simulink model "position_control"  (R2021a)
settings: Solver=ode23t  StartTime=0.0  StopTime=200  RelTol=1e-5
values from neighbouring files (symbols this model uses):
  g = 9.81    [quad_params.m]
  I = [     0.005831943165131                   0                   0 ... (first row only)    [quad_params.m]
  Kd_rates = [0.05,0.05,0.1]'    [quad_params.m]
  Kd_vel = [0.8,0.8,0.3]'    [quad_params.m]
  Ki_vel = [0.1,0.1,0.1]'    [quad_params.m]
  km = 1.2e-7    (= 1.2e-07)    [quad_params.m]
  Kp_att = [6,6,6]'    [quad_params.m]
  Kp_pos = [7,7,3]'    [quad_params.m]
  Kp_rates = [10,10,10]'    [quad_params.m]
  Kp_vel = [3,3,5]'    [quad_params.m]
  kt = 0.9e-5    (= 9e-06)    [quad_params.m]
  L = 0.2    [quad_params.m]
  m = 0.9272    [quad_params.m]
  q_init = [1;0;0;0]    [quad_params.m]
  rate_p_max = 3.5    [quad_params.m]
  thrust_max = thrust_max_per_motor*4    (= 32)    [quad_params.m]
  thrust_max_per_motor = 8    [quad_params.m]
  tilt_max = pi/6    (= 0.523598775598)    [quad_params.m]
  TQ_max_per_motor = km*(w_max.^2)    [quad_params.m]
  Vb_init = [0;0;0]    [quad_params.m]
  vel_xy_max = 15    [quad_params.m]
  vel_z_max = 10    [quad_params.m]
  wb_init = [0;0;0]    [quad_params.m]
  Xe_init = [0;0;0]    [quad_params.m]
undefined symbols (not defined in the file or in its folder): pm_0, sigbuilder_block, Vm_0, X, xme_0, Y, Z
libraries: simulink_extras x16, nesl_utility x5, aerolibutil x4, sm_lib x4, simulink x3, pid_lib x3, sharedtransform x3, sharedutil x1, vrlib x1, aerolibanim x1
(part 3 of 3)

== system position_control/Trajectory command/Yaw Sine/yaw ==
  Demux : Demux  Tag=STV Demux
      settings: DisplayOption=none
  FromWs : FromWorkspace  Tag=STV FromWs  VariableName=tuvar
      SigBuilderData=|
      | common.afterFinalStr = 'Extrapolate'
      | common.sampleTime = 0
      | dataSet(1).timeRange = [0 200]
      | dataSet(1).name = 'small_steps'
      | dataSet(2).timeRange = [0 200]
      | dataSet(2).name = 'zStairs_xyConstVEL'
      | dataSet(3).timeRange = [0 500]
      | dataSet(3).name = 'sineWaves'
      | dataSet(4).timeRange = [0 200]
      | dataSet(4).name = 'ZERO'
      | dataSet(5).timeRange = [0 200]
      | dataSet(5).name = 'SEARCH_P1'
      | sbobj.Name = 'Signal Builder'
      | sbobj.Groups(1).Name = 'small_steps'
      | sbobj.Groups(1).Signals(1).Name = 'Z'
      | sbobj.Groups(1).Signals(1).XData = [0 10 10.000001 20 20.000001 30 30.000001 55 200]
      | sbobj.Groups(1).Signals(1).YData = [0 0 2 2 2 2 2 2 2]
      | sbobj.Groups(1).Signals(2).Name = 'Y'
      | sbobj.Groups(1).Signals(2).XData = [0 10 10.000001 20 20.000001 30 30.000001 55 200]
      | sbobj.Groups(1).Signals(2).YData = [0 0 0 0 3 3 3 3 3]
      | sbobj.Groups(1).Signals(3).Name = 'X'
      | sbobj.Groups(1).Signals(3).XData = [0 10 10.000001 20 20.000001 30 30.000001 55 200]
      | sbobj.Groups(1).Signals(3).YData = [0 0 0 0 0 0 1 1 1]
      | sbobj.Groups(1).Signals(4).Name = 'Yaw'
      | sbobj.Groups(1).Signals(4).XData = [0 200]
      | sbobj.Groups(1).Signals(4).YData = [0 0]
      | sbobj.Groups(1).TimeRange = [0 200]
      | sbobj.Groups(2).Name = 'zStairs_xyConstVEL'
      | sbobj.Groups(2).Signals(1).Name = 'Z'
      | sbobj.Groups(2).Signals(1).XData = [0 10 10.000001 20 20.000001 30 30.000001 40 40.000001 55 200]
      | sbobj.Groups(2).Signals(1).YData = [0 0 1 1 2 2 1 1 0 0 0]
      | sbobj.Groups(2).Signals(2).Name = 'Y'
      | sbobj.Groups(2).Signals(2).XData = [0 10 10.000001 20 20.000001 30 30.000001 40 40.000001 55 200]
      | sbobj.Groups(2).Signals(2).YData = [0 1 1.0000001 2 2.0000001 3 3.0000001 4 4.0000001 5.5 20]
      | sbobj.Groups(2).Signals(3).Name = 'X'
      | sbobj.Groups(2).Signals(3).XData = [0 10 10.000001 20 20.000001 30 30.000001 40 40.000001 55 200]
      | sbobj.Groups(2).Signals(3).YData = [0 0.5 0.50000005 1 1.00000005 1.5 1.50000005 2 2.00000005 2.75 10]
      | sbobj.Groups(2).Signals(4).Name = 'Yaw'
      | sbobj.Groups(2).Signals(4).XData = [0 200]
      | sbobj.Groups(2).Signals(4).YData = [0 0]
      | sbobj.Groups(2).TimeRange = [0 200]
      | sbobj.Groups(3).Name = 'sineWaves'
      | sbobj.Groups(3).Signals(1).Name = 'Z'
      | sbobj.Groups(3).Signals(1).XData = [0 0.1 0.2 0.3 0.4 0.5 0.6 0.7 0.8 0.9 1 1.1 ... (5001 elements, 1x5001)]
      | sbobj.Groups(3).Signals(1).YData = [0 0.0314107325553 0.0627904665622 0.0941082340641 0.125333128258 0.156434333994 0.18738115819 0.218143060119 0.248689681547 0.278990876699 0.309016742004 0.338737645607 ... (5001 elements, 1x5001)]
      | sbobj.Groups(3).Signals(2).Name = 'Y'
      | sbobj.Groups(3).Signals(2).XData = [0 0.1 0.2 0.3 0.4 0.5 0.6 0.7 0.8 0.9 1 1.1 ... (5001 elements, 1x5001)]
      | sbobj.Groups(3).Signals(2).YData = [0 0.01 0.02 0.03 0.04 0.05 0.06 0.07 0.08 0.09 0.1 0.11 ... (5001 elements, 1x5001)]
      | sbobj.Groups(3).Signals(3).Name = 'X'
      | sbobj.Groups(3).Signals(3).XData = [0 0.1 0.2 0.3 0.4 0.5 0.6 0.7 0.8 0.9 1 1.1 ... (5001 elements, 1x5001)]
      | sbobj.Groups(3).Signals(3).YData = [0 0.0157073040455 0.0314107325553 0.04710641095 0.0627904665622 0.0784590295926 0.0941082340641 0.109734218776 0.125333128258 0.140901113717 0.156434333994 0.171928956505 ... (5001 elements, 1x5001)]
      | sbobj.Groups(3).Signals(4).Name = 'Yaw'
      | sbobj.Groups(3).Signals(4).XData = [0 500]
      | sbobj.Groups(3).Signals(4).YData = [0 0]
      | sbobj.Groups(3).TimeRange = [0 500]
      | sbobj.Groups(4).Name = 'ZERO'
      | sbobj.Groups(4).Signals(1).Name = 'Z'
      | sbobj.Groups(4).Signals(1).XData = [0 200]
      | sbobj.Groups(4).Signals(1).YData = [0 0]
      | sbobj.Groups(4).Signals(2).Name = 'Y'
      | sbobj.Groups(4).Signals(2).XData = [0 200]
      | sbobj.Groups(4).Signals(2).YData = [0 0]
      | sbobj.Groups(4).Signals(3).Name = 'X'
      | sbobj.Groups(4).Signals(3).XData = [0 200]
      | sbobj.Groups(4).Signals(3).YData = [0 0]
      | sbobj.Groups(4).Signals(4).Name = 'Yaw'
      | sbobj.Groups(4).Signals(4).XData = [0 200]
      | sbobj.Groups(4).Signals(4).YData = [0 0]
      | sbobj.Groups(4).TimeRange = [0 200]
      | sbobj.Groups(5).Name = 'SEARCH_P1'
      | sbobj.Groups(5).Signals(1).Name = 'Z'
      | sbobj.Groups(5).Signals(1).XData = [0 9.9 200]
      | sbobj.Groups(5).Signals(1).YData = [0 0 0]
      | sbobj.Groups(5).Signals(2).Name = 'Y'
      | sbobj.Groups(5).Signals(2).XData = [0 200]
      | sbobj.Groups(5).Signals(2).YData = [0 0]
      | sbobj.Groups(5).Signals(3).Name = 'X'
      | sbobj.Groups(5).Signals(3).XData = [0 200]
      | sbobj.Groups(5).Signals(3).YData = [0 0]
      | sbobj.Groups(5).Signals(4).Name = 'Yaw'
      | sbobj.Groups(5).Signals(4).XData = [0 0.689655172414 1.37931034483 2.06896551724 2.75862068966 3.44827586207 4.13793103448 4.8275862069 5.51724137931 6.20689655172 6.89655172414 7.58620689655 ... (291 elements, 1x291)]
      | sbobj.Groups(5).Signals(4).YData = [0 0.644911320633 1.25966730468 1.81552264558 2.28648616538 2.65053613334 2.89064997756 2.99560024155 2.96047956762 2.78693015945 2.48306699447 2.06309837656 ... (291 elements, 1x291)]
      | sbobj.Groups(5).TimeRange = [0 200]
  Z : Outport  VectorParamsAs1DForOutWhenUnconnected=off
  Y : Outport  Tag=STV Outport  Port=2  VectorParamsAs1DForOutWhenUnconnected=off
  X : Outport  Tag=STV Outport  Port=3  VectorParamsAs1DForOutWhenUnconnected=off
  Yaw : Outport  Tag=STV Outport  Port=4
  wires:
  Demux/4 -> Yaw/1
  Demux/3 -> X/1
  Demux/2 -> Y/1
  FromWs/1 -> Demux/1
  Demux/1 -> Z/1

== system position_control/Control allocation and motor control/Ideal Actuators with allocation/Control allocation/Subsystem ==
  w_per_sec : Inport
  Constant3 : Constant  Value=3.141592653589793
  Gain1 : Gain  Gain=2
  Product : Product  Inputs=*/
  RPS : Outport
  wires:
  Gain1/1 -> Product/2  "2PI"
  w_per_sec/1 -> Product/1
  Constant3/1 -> Gain1/1
  Product/1 -> RPS/1

== system position_control/Control allocation and motor control/Ideal Actuators with allocation/Control allocation/W2_checker ==
  w2_CMD : Inport
  Assertion{,1..3} (4 alike) : Assertion
  Compare To Constant : simulink/Logic and Bit Operations/Compare To Constant  relop=>=  const=0  OutDataTypeStr=boolean
  Demux : Demux
  w2 : Outport  VectorParamsAs1DForOutWhenUnconnected=off
  wires:
  w2_CMD/1 -> w2/1, Compare To Constant/1
  Compare To Constant/1 -> Demux/1
  Demux/1 -> Assertion/1
  Demux/4 -> Assertion3/1
  Demux/3 -> Assertion2/1
  Demux/2 -> Assertion1/1

== system position_control/Control allocation and motor control/Ideal Actuators with allocation/Perfect actuators/Motor Control ==
  w_CMD : Inport
  Demux : Demux
  Mux : Mux
  w CMD vs Actual : Scope  NumInputPorts=4
  w_MUX : Subsystem
  w : Outport  VectorParamsAs1DForOutWhenUnconnected=off
  wires:
  Demux/4 -> Mux/4
  Demux/3 -> Mux/3
  Demux/2 -> Mux/2
  Demux/1 -> Mux/1
  w_CMD/1 -> [W_CMD], Demux/1
  w_MUX/4(w4) -> w CMD vs Actual/4
  w_MUX/2(w2) -> w CMD vs Actual/2
  w_MUX/3(w3) -> w CMD vs Actual/3
  w_MUX/1(w1) -> w CMD vs Actual/1
  [W_CMD] -> w_MUX/1(W_CMD)
  Mux/1 -> w_MUX/2(W), w/1

== system position_control/Quad_EOM/Integrate_quaternion/NORMLIZE_occasionally/Adjust_to_UNITY ==
  note: Every 10 seconds normalize
      | the quaternion to ensure it is a
      | UNIT quaternion
  qin : Inport
  Data Type Conversion : DataTypeConversion  OutDataTypeStr=double
  Detect Increase : simulink/Logic and Bit Operations/Detect Increase  vinit=0.0  OutDataTypeStr=boolean
  MATLAB Function : MATLAB Function  TreatAsAtomicUnit=on
  Pulse Generator : DiscretePulseGenerator  PulseType=Time based  Period=10  PulseWidth=50
  Scope : Scope
  q_unit : Outport
  wires:
  Pulse Generator/1 -> Detect Increase/1
  Detect Increase/1 -> Data Type Conversion/1
  MATLAB Function/1(q) -> q_unit/1
  Data Type Conversion/1 -> MATLAB Function/1(change_signal)
  qin/1 -> MATLAB Function/2(q_in)
  MATLAB Function/2(mag_of_q) -> Scope/1

== system position_control/Control allocation and motor control/Ideal Actuators with allocation/Perfect actuators/Motor Control/w_MUX ==
  W_CMD : Inport
  W : Inport  Port=2
  Demux1 : Demux
  Demux2 : Demux
  Mux{,1..3} (4 alike) : Mux  Inputs=2
  w1 : Outport  VectorParamsAs1DForOutWhenUnconnected=off
  w2 : Outport  Port=2  VectorParamsAs1DForOutWhenUnconnected=off
  w3 : Outport  Port=3  VectorParamsAs1DForOutWhenUnconnected=off
  w4 : Outport  Port=4  VectorParamsAs1DForOutWhenUnconnected=off
  wires:
  W_CMD/1 -> Demux2/1
  W/1 -> Demux1/1
  Mux/1 -> w1/1
  Mux1/1 -> w2/1
  Mux3/1 -> w4/1
  Mux2/1 -> w3/1
  Demux2/1 -> Mux/1
  Demux2/2 -> Mux1/1
  Demux2/3 -> Mux2/1
  Demux2/4 -> Mux3/1
  Demux1/1 -> Mux/2
  Demux1/2 -> Mux1/2
  Demux1/3 -> Mux2/2
  Demux1/4 -> Mux3/2

== matlab function position_control/Quad_EOM/Integrate_quaternion/MATLAB Function2 ==
  data: R input; phi output; theta output; psi output
function [phi,theta,psi] = euler_from_rot(R)
% Get Euler angles from rotation matrix (wolrd to body rotation matrix)
%NOTE:  this is bRg ... and NOT gRb

phi   = atan2(R(2,3),R(3,3));
theta = -asin(R(1,3));
psi   = atan2(R(1,2), R(1,1));
end

== matlab function position_control/Thrust to attitude/Subsystem/MATLAB Function3 ==
  data: acc_w input size=[2 1]; phi_cmd output size=[2 1]; g input size=[1 1]; yaw_cmd input; theta_cmd output
function [phi_cmd,theta_cmd]= acc2ang(acc_w, g,yaw_cmd)
    
    phi_cmd = 1/g*(acc_w(1)*sin(yaw_cmd)-acc_w(2)*cos(yaw_cmd));
    theta_cmd = 1/g*(acc_w(1)*cos(yaw_cmd)+acc_w(2)*sin(yaw_cmd));
end

== matlab function position_control/Control allocation and motor control/Ideal Actuators with allocation/Perfect actuators/Allocation matrix (motor speed to twist) ==
  data: L input; Thrust output; kt input; km input; w2_col input; M_x output; M_y output; M_z output
function [Thrust, M_x, M_y, M_z] = mixer(L, kt, km, w2_col)
%#codegen



    % construct the co-efficient matrix:
    %  T = C * w^2
    
%     C = [
%         kt  ,   kt   ,   kt  ,   kt  ;
%         0   , -L*kt  ,   0   , L*kt  ;
%        L*kt ,   0    , -L*kt ,   0   ;
%         km ,   -km   ,  km  ,   -km  ;
%     ];

    C = [
        -kt  ,   -kt  ,   -kt ,   -kt  ;
        0    , -L*kt   ,   0   , L*kt  ;
       L*kt ,   0    , -L*kt  ,   0   ;
        -km  ,   km   ,  -km  ,   km  ;
    ];

    % solve for the FM_col
    %   FM_col = [Thrust, M_x, M_y, M_z].' ;
    
    FM_col  =  C * w2_col;
    
    Thrust  =  FM_col(1);
    M_x     =  FM_col(2);
    M_y     =  FM_col(3);
    M_z     =  FM_col(4);
    
end

== matlab function position_control/Quad_EOM/Integrate_quaternion/calc_bRg ==
  data: q input double size=[4, 1]; bRg output double size=[3 3]
function bRg = quat2dcm(q)
% convert quaternion to DCM
% the DCM represent coordinate transformation of a vector in inertial axes
% into body axes (bRg)

% VERY SLOW in SIMULINK

    q0    = q(1);
    qx    = q(2);
    qy    = q(3);
    qz    = q(4);
    
    C_11  = qx^2 + q0^2 - qy^2 - qz^2;
    C_12  = 2*(qx*qy + qz*q0);
    C_13  = 2*(qx*qz - qy*q0);
       
    C_21  = 2*(qx*qy - qz*q0);
    C_22  = qy^2 + q0^2 - qx^2 - qz^2;
    C_23  = 2*(qy*qz + qx*q0);
    
    C_31  = 2*(qx*qz + qy*q0);
    C_32  = 2*(qy*qz - qx*q0);
    C_33  = qz^2 + q0^2 - qx^2 - qy^2;
    
    
    bRg = [ C_11, C_12, C_13;
            C_21, C_22, C_23;
            C_31, C_32, C_33;   ];   


end

== matlab function position_control/Quad_EOM/Integrate_quaternion/calc_q_DOT ==
  data: q input double size=[4, 1]; q_dot output double size=[4 1]; wb input double size=[3, 1]
function q_dot = q_dot_from_rates(q, wb)
% angular rates are related to quaternion derivative by:
% note: this transformation is in body-fixed frame (body rates and
% quaternion in body-fixed frame)
% q_dot  = 0.5 * W^T * wb;
% 
% W = 
%    [-q1,  q0,  q3, -q2]
%    [-q2, -q3,  q0,  q1]
%    [-q3,  q2, -q1,  q0]
% W_transpose = 
%             [-q1, -q2, -q3]
%             [ q0, -q3,  q2]
%             [ q3,  q0, -q1]
%             [-q2,  q1,  q0]

q0     = q(1);
q1     = q(2);
q2     = q(3);
q3     = q(4);

W_transpose =  [
                 -q1, -q2, -q3;
                  q0, -q3,  q2;
                  q3,  q0, -q1;
                 -q2,  q1,  q0;
                 ];

wb = wb(:);

q_dot  = 0.5 * W_transpose * wb;

end

== matlab function position_control/Thrust to attitude/Subsystem/MATLAB Function5 ==
  data: body_z input; thr_dir output; acc_sp input; g input; hover_thrust input; thr_mag output
function [thr_dir,thr_mag] = project_thrust(body_z,acc_sp,g, hover_thrust)
    % body_z is normalized acceleration pointing down
    % hover_thrust = m*g
    collective_thrust = acc_sp(3) * (hover_thrust/g) - hover_thrust; % T=(m*acc_cmd)-(mg)
	% Project thrust to planned body attitude
    tmp = dot([0,0,1]',body_z);
	collective_thrust = collective_thrust./tmp;
	thr_dir = body_z*collective_thrust;

    % thrust body setpoint is the norm of the thrust vector
    thr_mag = norm(thr_dir);
    
%     final_body_z = unit(body_z); % normalize body_z
%     
%     % vector of desired yaw direction in XY plane, rotated by PI/2
%     y_c = [-sin(yaw_sp), cos(yaw_sp), 0.0].';
%     % desired body_x axis, orthogonal to body_z
% 	body_x = cross(y_c,final_body_z);
%     
%    % keep nose to front while inverted upside down
% 	if (final_body_z(3) < 0.0
% 		body_x = -body_x;
%     end
%     body_x = unit(body_x); % normalize body_x
%     % desired body_y axis
%     body_y = mod(final_body_z,body_x);
%     
%     % fill rotation matrix and convert to quaternion
%     world_unit = [0,0,1]';
%     body_unit = body_z;
%     dot_product_unit = dot(body_unit,world_unit);
% 	angle = acos(dot_product_unit);
%     body_unit = cos(angle) * world_unit + sin(angle) * body_unit;

== matlab function position_control/Thrust to attitude/Subsystem/MATLAB Function6 ==
  data: acc_w input size=[2 1]; u1_thrust output size=[2 1]; g input size=[1 1]; m input
function u1_thrust = acc2thrust(acc_w, g,m)
    
    u1_thrust = m*g+acc_w(3);
end

== matlab function position_control/Quad_EOM/Integrate_quaternion/NORMLIZE_occasionally/Adjust_to_UNITY/MATLAB Function ==
  data: change_signal input double size=1; q output; q_in input double size=[4 1]; mag_of_q output
function [q, mag_of_q] = fcn(change_signal, q_in)

if(change_signal > 0.5)
    q = q_in / norm(q_in);
else
    q = q_in;
end

mag_of_q = norm(q);

end

== matlab function position_control/Thrust to attitude/Subsystem/MATLAB Function7 ==
  data: acc_w input size=[2 1]; phi_cmd output size=[2 1]; g input size=[1 1]; yaw_cmd input; theta_cmd output
function [phi_cmd,theta_cmd]= acc2ang(acc_w, g,yaw_cmd)
    
    phi_cmd = 1/g*(acc_w(1)*sin(yaw_cmd)-acc_w(2)*cos(yaw_cmd));
    theta_cmd = 1/g*(acc_w(1)*cos(yaw_cmd)+acc_w(2)*sin(yaw_cmd));
end

== matlab function position_control/Thrust to attitude/Subsystem/MATLAB Function8 ==
  data: thrust_vec input; q_sp output; heading_angle input
function q_sp = thrust2quat(thrust_vec,heading_angle)
% full attitude control using both thrust vector and desired yaw
    % inputs: thrust_vec, heading_angle
    % extracted from: ardupilot
    thrust_vec_unit = [0,0,1]';
    
    if norm(thrust_vec)^2<1e-15
        thrust_vec = thrust_vec_unit;
    else
        thrust_vec = unit(thrust_vec);  % or normalize(thrust_vec)
    end
    % the cross product of the desired and target thrust vector defines the rotation vector
    thrust_vec_cross = cross(thrust_vec_unit, thrust_vec);
    % the dot product is used to calculate the angle between the target and desired thrust vectors
    thrust_vec_angle = acos(dot(thrust_vec_unit, thrust_vec));
    % Normalize the thrust rotation vector
    thrust_vec_length = norm(thrust_vec_cross);
    if thrust_vec_length==0 
        thrust_vec_length = 1;
        thrust_vec_cross = thrust_vec_unit;
    end
    thrust_vec_dir = thrust_vec_cross/thrust_vec_length;
    
    % convert thrust_vec_cross and thrust_vec_angle to quaternion
    thrust_vec_quat = axang2quat([thrust_vec_dir.', thrust_vec_angle]);
    % yaw quaternion from heading_angle and [0,0,1]
    yaw_quat = axang2quat([[0.0, 0.0, 1.0], heading_angle]);
    
    % multiple both quats to get quat setpoint
    q_sp = quatmultiply(thrust_vec_quat,yaw_quat);

== matlab function position_control/Attitude control/MATLAB Function1 ==
  data: q0 input; y output
function y = sign(q0)
if q0>=0
    y = 1;
else
    y = -1;
end

== matlab function position_control/Control allocation and motor control/Ideal Actuators with allocation/Control allocation/FM_to_w2 ==
  data: L input; w2_cmd output; kt input; km input; Thrust input; M_x input; M_y input; M_z input
function w2_cmd = control_allocation(L, kt, km, Thrust, M_x, M_y, M_z)
%#codegen

    % construct the co-efficient matrix:
    %  F_and_M = C * w^2
    %
    % C = [
    %     kt  ,   kt   ,   kt  ,   kt  ;
    %     0   , -L*kt  ,   0   , L*kt  ;
    %    L*kt ,   0    , -L*kt ,   0   ;
    %     km ,   -km   ,  km  ,   -km  ;
    % ];

    % used Symbolic toolbox to compute inv(C)
%     C_inv = [
%                 1/(4*kt),          0 ,  1/(2*L*kt),  1/(4*km);
%                 1/(4*kt), -1/(2*L*kt),           0,  -1/(4*km); 
%                 1/(4*kt),          0 , -1/(2*L*kt),  1/(4*km);
%                 1/(4*kt), 1/(2*L*kt) ,          0 ,  -1/(4*km);
%              ];
         
    C_inv = [
             -1/(4*kt),            0,   1/(2*L*kt), -1/(4*km);
             -1/(4*kt),  -1/(2*L*kt),            0,  1/(4*km);
             -1/(4*kt),            0,  -1/(2*L*kt), -1/(4*km);
             -1/(4*kt),   1/(2*L*kt),            0,  1/(4*km);
            ];        
    % solve for the w^2 vec
    F_and_M_col = [Thrust, M_x, M_y, M_z].' ;

    w2_cmd = C_inv * F_and_M_col;
   
end

== matlab function position_control/Position+Velocity Control/Velocity PID Controller/MATLAB Function ==
  data: Tmax input; tilt_max input; Tx input; Tx output; Ty input; Tz input; Ty output
function [Tx, Ty] = limit_tilt( Tmax, tilt_max, Tx, Ty, Tz)
% horizontal thrust magnituide at max tilt angle
T_hor = abs(Tz)*tan(tilt_max);
% maximum availble horizontal thrust magnituide 
T_hor_max = sqrt(abs(Tmax^2-Tz^2));
% limit horizontal thrust magnituide to max available
T_hor = min(T_hor,T_hor_max);

% saturate horizonal thrust components Tx,Ty if exceed T_hor
if Tx^2+Ty^2 > T_hor
   T_xy = norm([Tx,Ty]);
   Tx = (Tx/T_xy)*T_hor;
   Ty = (Ty/T_xy)*T_hor;

else
   Tx = Tx;
   Ty = Ty;

end

== matlab function position_control/Thrust to attitude/MATLAB Function4 ==
  data: thrust_sp input; R_sp output; yaw_sp input; thrust_mag output
function [R_sp,thrust_mag] = thurst2attitude(thrust_sp, yaw_sp)
% Create Full Desired Quaternion Based on Thrust Setpoint and Desired Yaw Angle
% from px4
    % Desired body_z axis direction
    body_z = -thrust_sp/norm(thrust_sp);

    % Vector of desired Yaw direction in XY plane, rotated by pi/2 (fake body_y axis)
    y_C = [-sin(yaw_sp), cos(yaw_sp), 0.0].';

    % Desired body_x axis direction
    body_x = cross(y_C, body_z);
    body_x = body_x/norm(body_x); % normalize

    % Desired body_y axis direction
    body_y = cross(body_z, body_x);

    % Desired rotation matrix
    R_sp = [body_x, body_y, body_z].';

    thrust_mag = -norm(thrust_sp);

== matlab function position_control/Thrust to attitude/Subsystem/MATLAB Function ==
  data: dcm input; cur_thrust_z output
function cur_thrust_z = dur_thrust_dir(dcm)

cur_thrust_z = dcm(:,3);

== matlab function position_control/Quad_EOM/Integrate_quaternion/Calc Euler_rates/euler_rates ==
  data: phi_t input; euler_rates output; theta_t input; p input; q input; r input
function euler_rates = euler_rates(phi_t,theta_t,p,q,r)
%#codegen

%    This function was generated by the Symbolic Math Toolbox version 8.7.
%    04-Nov-2022 08:55:55

euler_rates = [(p.*cos(theta_t)+r.*cos(phi_t).*sin(theta_t)+q.*sin(phi_t).*sin(theta_t))./cos(theta_t);q.*cos(phi_t)-r.*sin(phi_t);(r.*cos(phi_t)+q.*sin(phi_t))./cos(theta_t)];

== matlab function position_control/Thrust to attitude/Subsystem/MATLAB Function1 ==
  data: acc_w input; acc_b output; yaw input
function acc_b = fcn(acc_w,yaw)
    bRg = [  cos(yaw),  sin(yaw);
            -sin(yaw),  cos(yaw);

          ];  

    acc_b = bRg * acc_w;

== matlab function position_control/Thrust to attitude/Subsystem/MATLAB Function2 ==
  data: acc_w input size=[2 1]; u1_thrust output size=[2 1]; g input size=[1 1]; m input
function u1_thrust = acc2thrust(acc_w, g,m)
    
    u1_thrust = m*g+acc_w(3);
end
